simulink model "SingoloSerbatoio"  (R2022b)
settings: Solver=VariableStepAuto  StartTime=0.0  StopTime=30  RelTol=1e-3
values from neighbouring files (symbols this model uses):
  C = 10    [SingoloSerbatoioValues.m]
  g = 9.81    [SingoloSerbatoioValues.m]
  Q1 = 10    [SingoloSerbatoioValues.m]
  Q2 = 5    [SingoloSerbatoioValues.m]
  R = 1    [SingoloSerbatoioValues.m]
  ro = 1000    [SingoloSerbatoioValues.m]
settings Model: Creator=giuli  LastModifiedBy=giuli

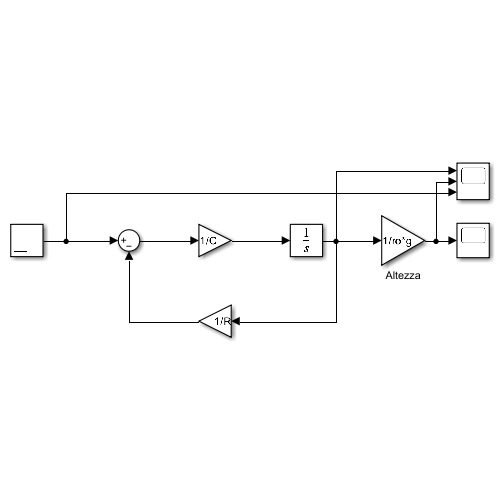
[thumbnail: Simulink's stored preview of the top-level diagram]
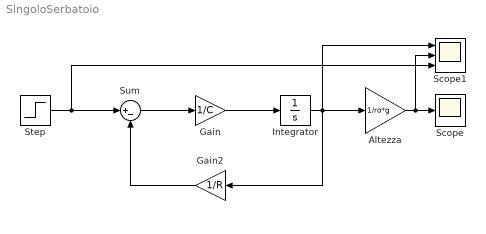
== system SingoloSerbatoio ==
  Altezza : Gain  Gain=1/ro*g
  Gain : Gain  Gain=1/C
  Gain2 : Gain  Gain=1/R
  Integrator : Integrator
  Scope : Scope
  Scope1 : Scope  NumInputPorts=3
  Step : Step  Time=10  Before=Q1  After=Q2  SampleTime=0
  Sum : Sum  Inputs=|+-
  wires:
  Gain/1 -> Integrator/1
  Sum/1 -> Gain/1
  Step/1 -> Scope1/3, Sum/1
  Integrator/1 -> Scope1/1, Gain2/1, Altezza/1
  Gain2/1 -> Sum/2
  Altezza/1 -> Scope1/2, Scope/1
